simulink model "Modello_estetico"  (Simulink 7.8)
settings: Solver=ode45  StartTime=0.0  StopTime=10.0  RelTol=1e-3
settings Model: Creator=Adriano  LastModifiedBy=Adriano

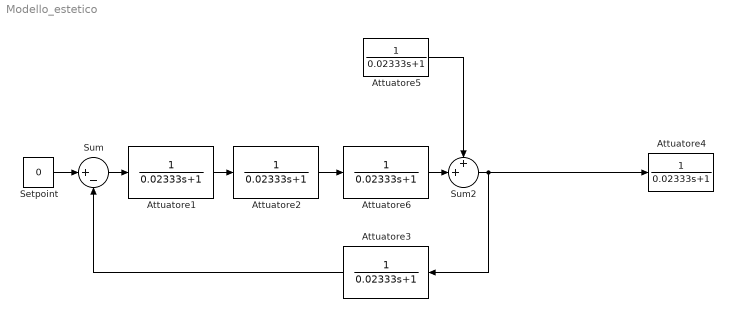
== system Modello_estetico ==
  Attuatore{1..6} (6 alike) : TransferFcn  Denominator=[0.02333 1]
  Setpoint : Constant  Value=0
  Sum : Sum  Inputs=|+-
  Sum2 : Sum  Inputs=++|
  wires:
  Setpoint/1 -> Sum/1
  Attuatore1/1 -> Attuatore2/1
  Attuatore2/1 -> Attuatore6/1
  Sum/1 -> Attuatore1/1
  Attuatore6/1 -> Sum2/2
  Sum2/1 -> Attuatore4/1, Attuatore3/1
  Attuatore3/1 -> Sum/2
  Attuatore5/1 -> Sum2/1
